simulink model "sampleModel1539"  (R2023a)
settings: Solver=VariableStepAuto  StartTime=0.0  StopTime=10.0  RelTol=1e-3
libraries: hdlsllib x4
settings Model: Creator=user1  LastModifiedBy=user1

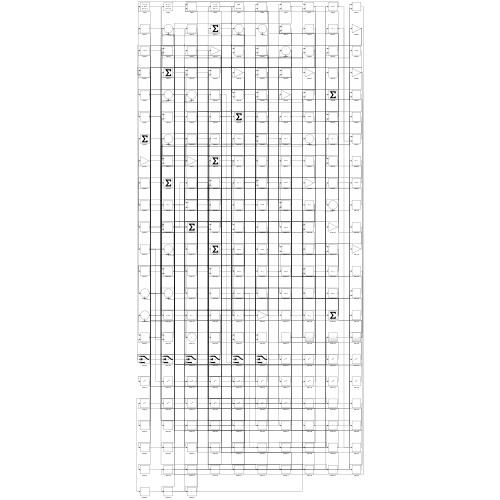
[thumbnail: Simulink's stored preview of the top-level diagram]
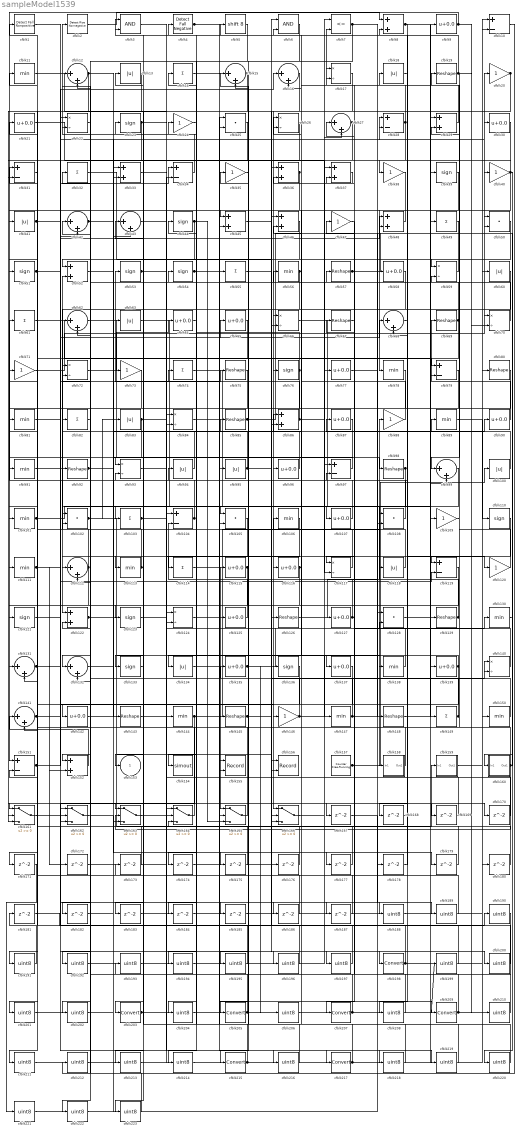
== system sampleModel1539 ==
  cfblk1 : hdlsllib/Logic and Bit Operations/Detect Fall Nonpositive  vinit=0  OutDataTypeStr=boolean
  cfblk{10,28,31,34,79,97,104,119,151} (9 alike) : Sum  Inputs=+-
  cfblk{13,18,41,60,63,83,94..95,100,118,134} (11 alike) : Abs  SaturateOnIntegerOverflow=off
  cfblk{11,56,78,81,89,91,101,106,111,113,130,138,144,147,150} (15 alike) : MinMax
  cfblk{25,50,102,105,108,128} (6 alike) : DotProduct  OutDataTypeStr=Inherit: Inherit via internal rule
  cfblk{14,32,49,55,61,74,82,103,114,149} (10 alike) : Sum  Inputs=+
  cfblk{9,21,30,58,64..65,77,87,90,96,107,115..116,125,127,135,137,139,142} (19 alike) : Bias  Bias=0.0  SaturateOnIntegerOverflow=off
  cfblk{20,24,35,38,40,47,71,73,88,109,120,146} (12 alike) : Gain
  cfblk{23,39,44,51,53..54,76,110,121,123,133,136} (12 alike) : Signum
  cfblk{12,15..16,27,42..43,62,68,99,112,131..132,141} (13 alike) : Sum  Inputs=|++
  cfblk{17,22,26,59,66,70,72,84,93,117,124,140} (12 alike) : Product  Inputs=*/  RndMeth=Zero  SaturateOnIntegerOverflow=on
  cfblk{8,29,33,36..37,45..46,48,52,86,122,152} (12 alike) : Sum
  cfblk{19,57,67,69,75,80,85,92,98,126,129,143,145,148} (14 alike) : Reshape
  cfblk154 : ToWorkspace  VariableName=simout  SaveFormat=Timeseries  SampleTime=-1
  cfblk155 : Record  FileSettingsInternal="{\"entries\":[{\"content\":{\"excelSettings\":{\"content\":{},\"type\":\"Streamout.ExcelSettings\"}},\"type\":\"Streamout.FileSettingStorage\",\"uuid\":\"\"}],\"packageUris\":[\"http:\\/\\/schema.mathworks.com\\/mf0\\/streamout_blocks\\/R2020a\"],\"version\":\"1.0\"}"  Layout=[1 1]  SignalsInternal="{\"entries\":[{\"content\":{\"signals\":[{\"content\":{\"blockPath\":[],\"dimensions\":[1],\"domain\":\"\",\"lineColor\":\"#a2142f\",\"plots\":[1],\"port\":1,\"signalID\":1573,\"signalName\":\"XY Graph:1\"},\"type\":\"RecordBlkView.Signal\",\"uuid\":\"\"},{\"content\":{\"blockPath\":[],\"dimensions\":[1],\"domain\":\"\",\"lineColor\":\"#139fff\",\"plots\":[1],\"port\":2,\"signalID\":1576,\"signalName\":\"XY Graph:2\"},\"type\":\"RecordBlkView.Signal\",\"uuid\":\"\"}]},\"type\":\"RecordBlkView.InputSignals\",\"uuid\":\"\"}],\"packageUris\":[\"http:\\/\\/schema.mathworks.com\\/mf0\\/streamout_blocks\\/R2020a\"],\"version\":\"1.0\"}"  VisualizationBindings="{\"xyplotplugin\":{\"info\":[{\"series\":[{\"bindingParametersList\":[{\"parameter\":\"X-Axis\",\"signalID\":1573,\"signalName\":\"XY Graph:1\"},{\"parameter\":\"Y-Axis\",\"signalID\":1576,\"signalName\":\"XY Graph:2\"}],\"seriesID\":20089}],\"subplotID\":1}]}}"  CompatibilityTag=XY  st=-1
  cfblk156 : Record  FileSettingsInternal="{\"entries\":[{\"content\":{\"excelSettings\":{\"content\":{},\"type\":\"Streamout.ExcelSettings\"}},\"type\":\"Streamout.FileSettingStorage\",\"uuid\":\"\"}],\"packageUris\":[\"http:\\/\\/schema.mathworks.com\\/mf0\\/streamout_blocks\\/R2020a\"],\"version\":\"1.0\"}"  Layout=[1 1]  SignalsInternal="{\"entries\":[{\"content\":{\"signals\":[{\"content\":{\"blockPath\":[],\"dimensions\":[1],\"domain\":\"\",\"lineColor\":\"#a2142f\",\"plots\":[1],\"port\":1,\"signalID\":1581,\"signalName\":\"XY Graph:1\"},\"type\":\"RecordBlkView.Signal\",\"uuid\":\"\"},{\"content\":{\"blockPath\":[],\"dimensions\":[1],\"domain\":\"\",\"lineColor\":\"#139fff\",\"plots\":[1],\"port\":2,\"signalID\":1584,\"signalName\":\"XY Graph:2\"},\"type\":\"RecordBlkView.Signal\",\"uuid\":\"\"}]},\"type\":\"RecordBlkView.InputSignals\",\"uuid\":\"\"}],\"packageUris\":[\"http:\\/\\/schema.mathworks.com\\/mf0\\/streamout_blocks\\/R2020a\"],\"version\":\"1.0\"}"  VisualizationBindings="{\"xyplotplugin\":{\"info\":[{\"series\":[{\"bindingParametersList\":[{\"parameter\":\"X-Axis\",\"signalID\":1581,\"signalName\":\"XY Graph:1\"},{\"parameter\":\"Y-Axis\",\"signalID\":1584,\"signalName\":\"XY Graph:2\"}],\"seriesID\":3946}],\"subplotID\":1}]}}"  CompatibilityTag=XY  st=-1
  cfblk157 : hdlsllib/Sources/Counter Free-Running  NumBits=16  tsamp=-1
  cfblk158 : Subsystem
      settings: LibrarySourceBlock=|
      | hdlsllib/Ports &
      | Subsystems/Subsystem
  cfblk159 : Subsystem
      settings: LibrarySourceBlock=|
      | hdlsllib/Ports &
      | Subsystems/Subsystem
  cfblk160 : Subsystem
      settings: LibrarySourceBlock=|
      | hdlsllib/Ports &
      | Subsystems/Subsystem
  cfblk{161..166} (6 alike) : Switch  SaturateOnIntegerOverflow=off  InputSameDT=off
  cfblk{167..187} (21 alike) : Delay  SampleTime=1
  cfblk{188..197,199..202,204,206,208,210..214,216,218..223} (29 alike) : DataTypeConversion  OutDataTypeStr=uint8  SaturateOnIntegerOverflow=off  RndMeth=Floor
  cfblk{198,203,205,207,209,215,217} (7 alike) : DataTypeConversion  SaturateOnIntegerOverflow=off  RndMeth=Floor
  cfblk2 : hdlsllib/Logic and Bit Operations/Detect Rise Nonnegative  vinit=0  OutDataTypeStr=boolean
  cfblk3 : Logic  AllPortsSameDT=off  OutDataTypeStr=boolean
  cfblk4 : hdlsllib/Logic and Bit Operations/Detect Fall Negative  vinit=0  OutDataTypeStr=boolean
  cfblk5 : ArithShift  BitShiftNumber=8
  cfblk6 : Logic  AllPortsSameDT=off  OutDataTypeStr=boolean
  cfblk7 : RelationalOperator  Operator=<=  OutDataTypeStr=boolean  InputSameDT=off
  cfblk153 : Outport  VectorParamsAs1DForOutWhenUnconnected=off
  wires:
  cfblk51/1 -> cfblk196/1, cfblk216/1
  cfblk40/1 -> cfblk78/1, cfblk160/1(In1), cfblk38/1
  cfblk46/1 -> cfblk166/1
  cfblk28/1 -> cfblk5/1, cfblk164/2, cfblk161/2
  cfblk101/1 -> cfblk107/1, cfblk48/2
  cfblk102/1 -> cfblk159/1(In1), cfblk145/1, cfblk83/1
  cfblk157/1 -> cfblk100/1, cfblk140/1
  cfblk59/1 -> cfblk52/1
  cfblk56/1 -> cfblk122/1, cfblk26/2
  cfblk17/1 -> cfblk116/1
  cfblk68/1 -> cfblk117/1
  cfblk9/1 -> cfblk151/1, cfblk210/1
  cfblk149/1 -> cfblk32/1, cfblk17/1, cfblk118/1
  cfblk41/1 -> cfblk162/1, cfblk16/1
  cfblk114/1 -> cfblk165/1
  cfblk107/1 -> cfblk61/1
  cfblk112/1 -> cfblk131/1, cfblk21/1
  cfblk85/1 -> cfblk48/1, cfblk197/1
  cfblk80/1 -> cfblk111/1
  cfblk91/1 -> cfblk52/2
  cfblk53/1 -> cfblk123/1, cfblk218/1
  cfblk61/1 -> cfblk76/1
  cfblk164/1 -> cfblk71/1
  cfblk2/1 -> cfblk8/1
  cfblk145/1 -> cfblk46/1, cfblk140/2
  cfblk20/1 -> cfblk131/2, cfblk174/1
  cfblk7/1 -> cfblk120/1, cfblk194/1
  cfblk70/1 -> cfblk18/1
  cfblk115/1 -> cfblk15/2, cfblk184/1, cfblk202/1
  cfblk125/1 -> cfblk104/2
  cfblk117/1 -> cfblk62/1
  cfblk19/1 -> cfblk99/1, cfblk3/2, cfblk70/2
  cfblk14/1 -> cfblk217/1
  cfblk139/1 -> cfblk134/1, cfblk204/1
  cfblk118/1 -> cfblk44/1
  cfblk66/1 -> cfblk149/1
  cfblk83/1 -> cfblk93/1, cfblk186/1, cfblk187/1
  cfblk37/1 -> cfblk36/2
  cfblk71/1 -> cfblk20/1
  cfblk148/1 -> cfblk9/1
  cfblk57/1 -> cfblk40/1, cfblk17/2
  cfblk62/1 -> cfblk165/2
  cfblk23/1 -> cfblk98/1, cfblk191/1
  cfblk8/1 -> cfblk109/1, cfblk68/2
  cfblk49/1 -> cfblk203/1
  cfblk126/1 -> cfblk58/1
  cfblk50/1 -> cfblk59/1
  cfblk120/1 -> cfblk19/1
  cfblk88/1 -> cfblk56/1
  cfblk22/1 -> cfblk132/1
  cfblk106/1 -> cfblk205/1
  cfblk165/1 -> cfblk13/1
  cfblk34/1 -> cfblk2/1
  cfblk63/1 -> cfblk105/1
  cfblk47/1 -> cfblk207/1
  cfblk74/1 -> cfblk158/1(In1)
  cfblk113/1 -> cfblk11/1, cfblk93/2
  cfblk150/1 -> cfblk94/1
  cfblk3/1 -> cfblk124/1
  cfblk31/1 -> cfblk161/1
  cfblk86/1 -> cfblk53/1, cfblk27/2
  cfblk73/1 -> cfblk152/1
  cfblk163/1 -> cfblk130/1
  cfblk4/1 -> cfblk55/1, cfblk79/1
  cfblk15/1 -> cfblk153/1, cfblk45/2
  cfblk134/1 -> cfblk95/1
  cfblk48/1 -> cfblk41/1
  cfblk77/1 -> cfblk148/1
  cfblk142/1 -> cfblk166/2
  cfblk104/1 -> cfblk3/1, cfblk102/1
  cfblk89/1 -> cfblk110/1
  cfblk38/1 -> cfblk66/1
  cfblk32/1 -> cfblk126/1
  cfblk135/1 -> cfblk39/1, cfblk206/1
  cfblk103/1 -> cfblk119/1, cfblk185/1
  cfblk158/1(Out1) -> cfblk31/1
  cfblk16/1 -> cfblk66/2
  cfblk92/1 -> cfblk85/1, cfblk70/1
  cfblk36/1 -> cfblk121/1, cfblk155/2
  cfblk35/1 -> cfblk215/1
  cfblk109/1 -> cfblk29/2
  cfblk21/1 -> cfblk97/1
  cfblk121/1 -> cfblk22/1
  cfblk44/1 -> cfblk133/1, cfblk165/3
  cfblk11/1 -> cfblk144/1
  cfblk100/1 -> cfblk87/1
  cfblk127/1 -> cfblk24/1, cfblk37/2
  cfblk39/1 -> cfblk103/1
  cfblk64/1 -> cfblk4/1
  cfblk60/1 -> cfblk72/1
  cfblk95/1 -> cfblk23/1, cfblk28/2
  cfblk12/1 -> cfblk63/1, cfblk162/3
  cfblk144/1 -> cfblk77/1, cfblk161/3
  cfblk67/1 -> cfblk137/1
  cfblk146/1 -> cfblk74/1, cfblk108/1
  cfblk84/1 -> cfblk209/1
  cfblk140/1 -> cfblk57/1
  cfblk122/1 -> cfblk147/1, cfblk28/1
  cfblk96/1 -> cfblk15/1
  cfblk55/1 -> cfblk156/1
  cfblk79/1 -> cfblk113/1
  cfblk54/1 -> cfblk166/3, cfblk138/1
  cfblk30/1 -> cfblk51/1
  cfblk128/1 -> cfblk129/1
  cfblk29/1 -> cfblk7/2
  cfblk152/1 -> cfblk141/1
  cfblk42/1 -> cfblk96/1, cfblk105/2
  cfblk159/1(Out1) -> cfblk80/1
  cfblk151/1 -> cfblk34/1, cfblk73/1
  cfblk132/1 -> cfblk90/1
  cfblk72/1 -> cfblk64/1
  cfblk138/1 -> cfblk27/1
  cfblk76/1 -> cfblk125/1, cfblk54/1
  cfblk27/1 -> cfblk117/2, cfblk45/1
  cfblk97/1 -> cfblk91/1
  cfblk24/1 -> cfblk114/1
  cfblk65/1 -> cfblk163/1
  cfblk5/1 -> cfblk142/1
  cfblk69/1 -> cfblk101/1, cfblk42/1
  cfblk13/1 -> cfblk31/2
  cfblk105/1 -> cfblk112/1
  cfblk111/1 -> cfblk146/1, cfblk152/2, cfblk75/1
  cfblk58/1 -> cfblk136/1
  cfblk147/1 -> cfblk86/1, cfblk50/2
  cfblk99/1 -> cfblk124/2
  cfblk129/1 -> cfblk88/1, cfblk16/2
  cfblk93/1 -> cfblk89/1
  cfblk108/1 -> cfblk62/2
  cfblk141/1 -> cfblk65/1, cfblk42/2
  cfblk94/1 -> cfblk12/1
  cfblk131/1 -> cfblk119/2, cfblk68/1, cfblk30/1, cfblk172/1
  cfblk90/1 -> cfblk69/1
  cfblk78/1 -> cfblk154/1
  cfblk98/1 -> cfblk112/2, cfblk182/1
  cfblk116/1 -> cfblk26/1, cfblk211/1
  cfblk52/1 -> cfblk143/1
  cfblk87/1 -> cfblk156/2
  cfblk81/1 -> cfblk198/1
  cfblk160/1(Out1) -> cfblk163/2, cfblk59/2, cfblk135/1, cfblk50/1
  cfblk124/1 -> cfblk167/1
  cfblk18/1 -> cfblk168/1
  cfblk168/1 -> cfblk8/2
  cfblk161/1 -> cfblk169/1
  cfblk169/1 -> cfblk7/1
  cfblk166/1 -> cfblk170/1
  cfblk170/1 -> cfblk104/1
  cfblk119/1 -> cfblk171/1
  cfblk172/1 -> cfblk34/2
  cfblk173/1 -> cfblk141/2
  cfblk174/1 -> cfblk86/2
  cfblk123/1 -> cfblk175/1
  cfblk175/1 -> cfblk22/2
  cfblk45/1 -> cfblk176/1
  cfblk176/1 -> cfblk72/2
  cfblk143/1 -> cfblk177/1
  cfblk177/1 -> cfblk122/2
  cfblk178/1 -> cfblk128/2
  cfblk162/1 -> cfblk179/1
  cfblk179/1 -> cfblk36/1
  cfblk180/1 -> cfblk102/2
  cfblk182/1 -> cfblk163/3
  cfblk137/1 -> cfblk183/1
  cfblk183/1 -> cfblk37/1
  cfblk184/1 -> cfblk29/1
  cfblk185/1 -> cfblk79/2
  cfblk186/1 -> cfblk132/2
  cfblk187/1 -> cfblk151/2
  cfblk1/1 -> cfblk188/1
  cfblk188/1 -> cfblk60/1
  cfblk167/1 -> cfblk189/1
  cfblk189/1 -> cfblk1/1
  cfblk181/1 -> cfblk190/1
  cfblk191/1 -> cfblk181/1
  cfblk25/1 -> cfblk192/1
  cfblk192/1 -> cfblk127/1
  cfblk190/1 -> cfblk193/1
  cfblk193/1 -> cfblk25/1
  cfblk194/1 -> cfblk25/2
  cfblk6/1 -> cfblk195/1
  cfblk195/1 -> cfblk173/1
  cfblk196/1 -> cfblk6/1
  cfblk197/1 -> cfblk6/2
  cfblk198/1 -> cfblk150/1, cfblk67/1
  cfblk199/1 -> cfblk81/1
  cfblk33/1 -> cfblk200/1
  cfblk200/1 -> cfblk162/2
  cfblk136/1 -> cfblk201/1
  cfblk201/1 -> cfblk33/1
  cfblk202/1 -> cfblk33/2
  cfblk203/1 -> cfblk199/1, cfblk115/1
  cfblk204/1 -> cfblk49/1
  cfblk205/1 -> cfblk12/2, cfblk92/1
  cfblk206/1 -> cfblk106/1
  cfblk207/1 -> cfblk99/2, cfblk164/1
  cfblk110/1 -> cfblk208/1
  cfblk208/1 -> cfblk47/1
  cfblk209/1 -> cfblk180/1, cfblk97/2
  cfblk210/1 -> cfblk84/1
  cfblk211/1 -> cfblk84/2
  cfblk10/1 -> cfblk212/1
  cfblk212/1 -> cfblk139/1
  cfblk133/1 -> cfblk213/1
  cfblk213/1 -> cfblk10/1
  cfblk75/1 -> cfblk214/1
  cfblk214/1 -> cfblk10/2
  cfblk215/1 -> cfblk108/2, cfblk155/1
  cfblk216/1 -> cfblk35/1
  cfblk217/1 -> cfblk164/3, cfblk46/2
  cfblk218/1 -> cfblk14/1
  cfblk43/1 -> cfblk219/1
  cfblk219/1 -> cfblk128/1
  cfblk130/1 -> cfblk220/1
  cfblk220/1 -> cfblk43/1
  cfblk171/1 -> cfblk221/1
  cfblk221/1 -> cfblk43/2
  cfblk82/1 -> cfblk222/1
  cfblk222/1 -> cfblk178/1
  cfblk26/1 -> cfblk223/1
  cfblk223/1 -> cfblk82/1

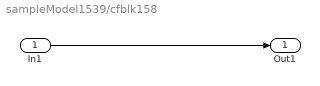
== system sampleModel1539/cfblk158 ==
  In1 : Inport
  Out1 : Outport
  wires:
  In1/1 -> Out1/1

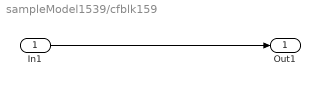
== system sampleModel1539/cfblk159 ==
  In1 : Inport
  Out1 : Outport
  wires:
  In1/1 -> Out1/1

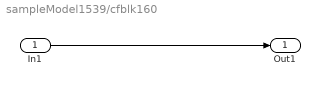
== system sampleModel1539/cfblk160 ==
  In1 : Inport
  Out1 : Outport
  wires:
  In1/1 -> Out1/1
